simulink model "sim11ex3"  (Simulink 2.09)
settings: Solver=ode45  StartTime=0.0  StopTime=3  MaxStep=.0250  RelTol=1e-3  AbsTol=1e-3
settings Model: SaveTime=off  SaveOutput=off  ConsistencyChecking=off  RTWTemplateMakefile=grt_vc.tmf

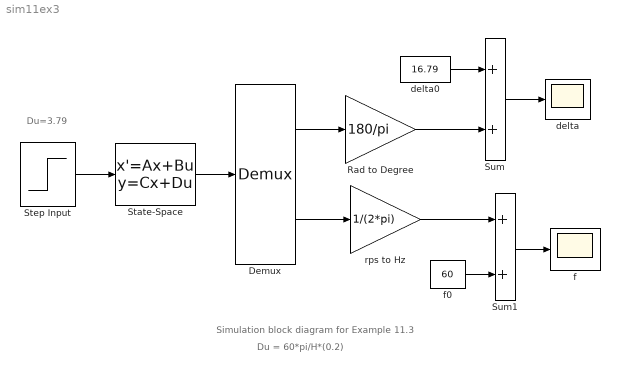
== system sim11ex3 ==
  note: Du=3.79
  note: Du = 60*pi/H*(0.2)
  note: Simulation block diagram for Example 11.3
  Demux : Demux  Outputs=2
  "Rad to Degree  " : Gain  Gain=180/pi
  State-Space : StateSpace  A="[0    1;  -37.7061   -2.6169 ]"  B="[0;   1]"  C=eye(2)  D=zeros(2, 1)  X0=0
  Step Input : Step  Time=100  Before=pi*60/9.94*.2  After=pi*60/9.84*.2
  Sum : Sum  Inputs=++
  Sum1 : Sum  Inputs=++
  delta : Scope
      settings: TickLabels=on  TimeRange=auto  YMin=-5  YMax=5  SaveToWorkspace=off  SaveName=ScopeData
  delta0 : Constant  Value=16.79
  f : Scope
      settings: TickLabels=on  TimeRange=auto  YMin=-5  YMax=5  SaveToWorkspace=off  SaveName=ScopeData
  f0 : Constant  Value=60
  rps to Hz : Gain  Gain=1/(2*pi)
  wires:
  f0/1 -> Sum1/2
  rps to Hz/1 -> Sum1/1
  delta0/1 -> Sum/1
  Demux/2 -> rps to Hz/1
  Sum/1 -> delta/1
  "Rad to Degree  "/1 -> Sum/2
  Demux/1 -> "Rad to Degree  "/1
  Sum1/1 -> f/1
  State-Space/1 -> Demux/1
  Step Input/1 -> State-Space/1
